simulink model "C172S_Longitudinal_OpenLoop"  (R2026a)
settings: Solver=ode4  StartTime=0  StopTime=40  FixedStep=0.01
InitFcn:
  | fcData = c172sLongitudinalData();
  | [~, fcPlant] = c172sLongitudinalPlant(fcData);
  | A_long = fcPlant.A; B_long = fcPlant.B;
  | C_long = fcPlant.C; D_long = fcPlant.D;
  | x0_long = zeros(4,1);
  | deltaE_step_rad = -deg2rad(1.0);
settings Model: Creator=Shahi  LastModifiedBy=Shahi

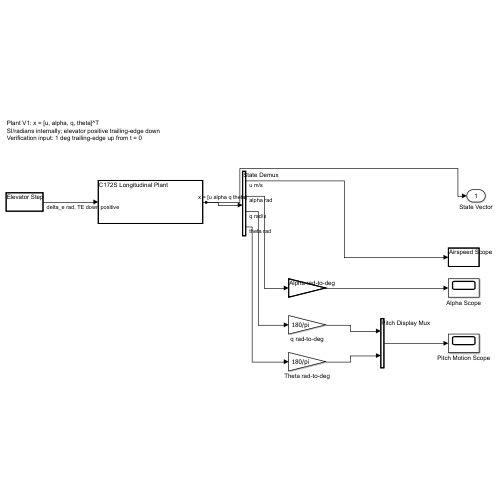
[thumbnail: Simulink's stored preview of the top-level diagram]
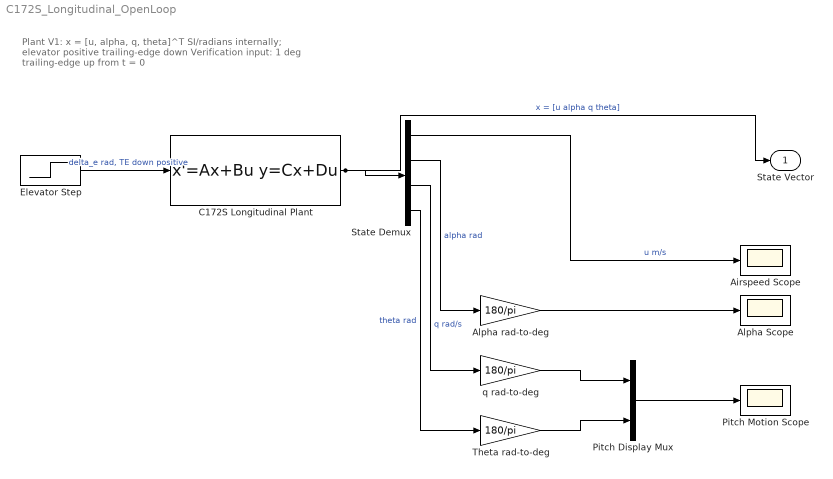
== system C172S_Longitudinal_OpenLoop ==
  note: Plant V1: x = [u, alpha, q, theta]^T
      | SI/radians internally; elevator positive trailing-edge down
      | Verification input: 1 deg trailing-edge up from t = 0
  Airspeed Scope : Scope
  Alpha Scope : Scope
  Alpha rad-to-deg : Gain  Gain=180/pi
  C172S Longitudinal Plant : StateSpace  A=A_long  B=B_long  C=C_long  D=D_long  InitialCondition=x0_long
  Elevator Step : Step  Time=0.0  InitialValue=0.0  FinalValue=deltaE_step_rad  SampleTime=0
  Pitch Display Mux : Mux  Inputs=2
  Pitch Motion Scope : Scope
  State Demux : Demux
  Theta rad-to-deg : Gain  Gain=180/pi
  q rad-to-deg : Gain  Gain=180/pi
  State Vector : Outport
  wires:
  Elevator Step/1 -> C172S Longitudinal Plant/1  "delta_e rad, TE down positive"
  C172S Longitudinal Plant/1 -> State Vector/1, State Demux/1  "x = [u alpha q theta]"
  State Demux/1 -> Airspeed Scope/1  "u m/s"
  State Demux/2 -> Alpha rad-to-deg/1  "alpha rad"
  Alpha rad-to-deg/1 -> Alpha Scope/1
  State Demux/3 -> q rad-to-deg/1  "q rad/s"
  q rad-to-deg/1 -> Pitch Display Mux/1
  State Demux/4 -> Theta rad-to-deg/1  "theta rad"
  Theta rad-to-deg/1 -> Pitch Display Mux/2
  Pitch Display Mux/1 -> Pitch Motion Scope/1
